simulink subsystem "controlStates"  (R2022b)
settings: Solver=VariableStepAuto  StartTime=0.0  StopTime=10.0  RelTol=1e-3
libraries: Raptor_lib x3
settings Model: Creator=serga  LastModifiedBy=serga

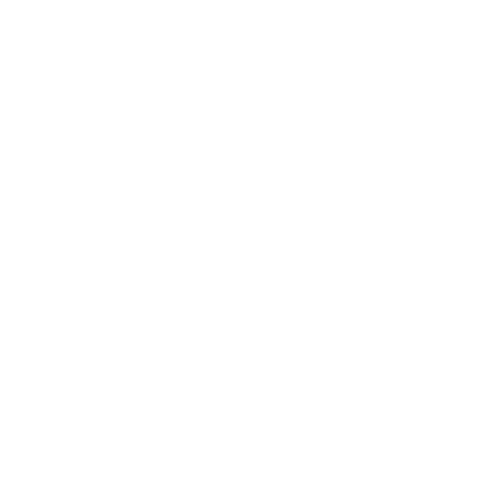
[thumbnail: Simulink's stored preview of the top-level diagram]
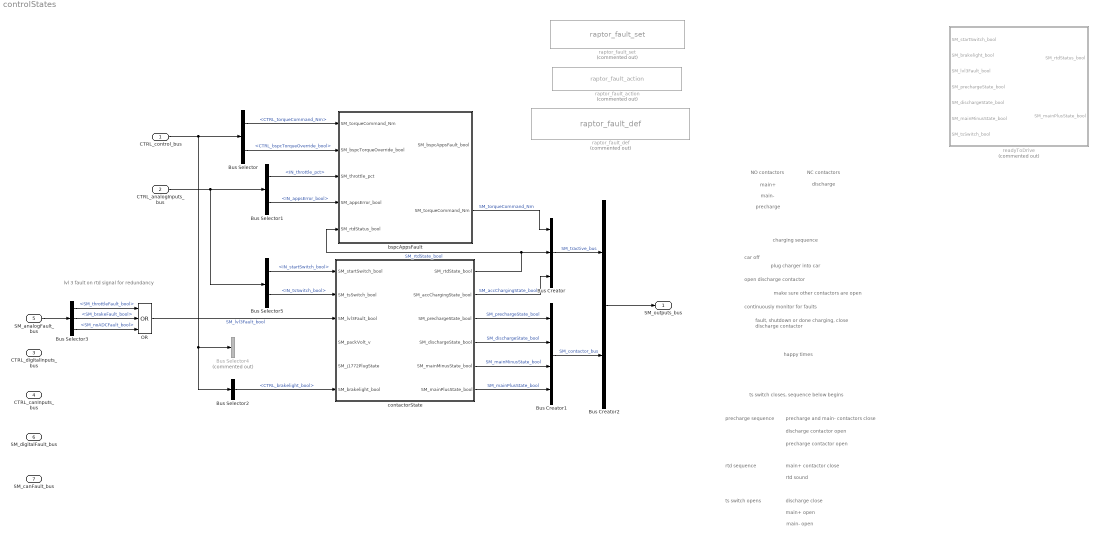
== system controlStates ==
  note: lvl 3 fault on rtd signal for redundancy
  note: ts switch closes, sequence below begins
  note: precharge sequence
  note: precharge and main- contactors close
  note: discharge contactor open
  note: NO contactors
  note: main+
  note: main-
  note: precharge
  note: precharge contactor open
  note: NC contactors
  note: discharge
  note: rtd sequence
  note: main+ contactor close
  note: rtd sound
  note: ts switch opens
  note: discharge close
  note: main+ open
  note: main- open
  note: charging sequence
  note: car off
  note: plug charger into car
  note: open discharge contactor
  note: continuously monitor for faults
  note: fault, shutdown or done charging, close discharge contactor
  note: happy times
  note: make sure other contactors are open
  CTRL_control_bus : Inport
  CTRL_analogInputs_bus : Inport  Port=2
  CTRL_digitalInputs_bus : Inport  Port=3
  CTRL_canInputs_bus : Inport  Port=4
  SM_analogFault_bus : Inport  Port=5
  SM_digitalFault_bus : Inport  Port=6
  SM_canFault_bus : Inport  Port=7
  Bus Creator : BusCreator  Inputs=3
  Bus Creator1 : BusCreator  Inputs=4
  Bus Creator2 : BusCreator  Inputs=2
  Bus Selector : BusSelector  OutputSignals=CTRL_tractive_bus.CTRL_torqueCommand_Nm,CTRL_tractive_bus.CTRL_bspcTorqueOverride_bool
  Bus Selector1 : BusSelector  OutputSignals=IN_throttle_bus.IN_throttle_pct,IN_throttle_bus.IN_appsError_bool
  Bus Selector2 : BusSelector  OutputSignals=CTRL_brake_bus.CTRL_brakelight_bool
  Bus Selector3 : BusSelector  OutputSignals=SM_lvl3AnalogFault_bus.SM_throttleFault_bool,SM_lvl3AnalogFault_bus.SM_brakeFault_bool,SM_lvl3AnalogFault_bus.SM_noADCFault_bool
  Bus Selector4 : BusSelector  Commented=on  OutputSignals=signal1,signal2
  Bus Selector5 : BusSelector  OutputSignals=IN_startSwitch_bus.IN_startSwitch_bool,IN_tsSwitch_bus.IN_tsSwitch_bool
  OR : Logic  Operator=OR  Inputs=3  IconShape=distinctive  AllPortsSameDT=off  OutDataTypeStr=boolean
  bspcAppsFault : Stateflow chart  TreatAsAtomicUnit=on
      settings: PortSchema="{\"entries\":[{\"content\":{\"sides\":[{\"content\":{\"connectorIds\":[\"In1\",\"In2\",\"In5\",\"In3\",\"In4\"]},\"type\":\"ConnectorPlacement.EquallySpacedRectSide\",\"uuid\":\"848a0214-b289-4fde-8f30-558c176c1664\"},{\"content\":{\"connectorIds\":[\"Out1\",\"Out2\"],\"side\":\"RIGHT\"},\"type\":\"ConnectorPlacement.EquallySpacedRectSide\",\"uuid\":\"0594a9c2-6fff-42f9-9aad-f57b5a6a5f51\"},{\"content\":{\"connectorIds\":[],\"side\":\"TOP\"},\"type\":\"ConnectorPlacement.EquallySpacedRectSide\",\"uuid\":\"66d9e814-45e9-4ebd-81f9-9e1bbba2abf2\"}]},\"type\":\"ConnectorPlacement.EquallySpacedConnector\",\"uuid\":\"77a7b6c4-8b57-4880-abaf-81cbc3ed0df8\"}],\"packageUris\":[\"http://schema.mathworks.com/mf0/Connector/R2020b\"],\"version\":\"1.0\"}"
  contactorState : Stateflow chart  TreatAsAtomicUnit=on
      settings: PortSchema="{\"entries\":[{\"content\":{\"sides\":[{\"content\":{\"connectorIds\":[\"In5\",\"In1\",\"In3\",\"In2\",\"In4\",\"In6\"]},\"type\":\"ConnectorPlacement.EquallySpacedRectSide\",\"uuid\":\"5a1b01df-5f74-4071-b1de-8ca561e5e723\"},{\"content\":{\"connectorIds\":[\"Out4\",\"Out6\",\"Out1\",\"Out2\",\"Out3\",\"Out5\"],\"side\":\"RIGHT\"},\"type\":\"ConnectorPlacement.EquallySpacedRectSide\",\"uuid\":\"0ef1ebc5-2a8c-458a-b0e0-8c2b473d38b4\"},{\"content\":{\"connectorIds\":[],\"side\":\"TOP\"},\"type\":\"ConnectorPlacement.EquallySpacedRectSide\",\"uuid\":\"5065868a-8688-4951-998e-140db11ca85e\"}]},\"type\":\"ConnectorPlacement.EquallySpacedConnector\",\"uuid\":\"42e1f654-1cfc-4608-be09-c21f3bede254\"}],\"packageUris\":[\"http://schema.mathworks.com/mf0/Connector/R2020b\"],\"version\":\"1.0\"}"
  raptor_fault_action : Raptor_lib/Faults/raptor_fault_action  Commented=on  actionName='myFaultAction'  calVisible=off  calAccess=1  calFunction='System | FaultManager | FaultAction'
      settings: SourceProductName=Raptor
  raptor_fault_def : Raptor_lib/Faults/raptor_fault_def  Commented=on  faultName='SM_bspcAppsFault_bool'  persist=off  sticky=off  emisRelated=off  singleTrip=off  clearMethod=Standard  xLimit=25  yLimit=50  calEnable=on  addDisable=off  calAccess=1  calFunction='System | FaultManager'
      settings: SourceProductName=Raptor
  raptor_fault_set : Raptor_lib/Faults/raptor_fault_set  Commented=on  faultSourceValues=[]  faultSource=2  faultName='myFault'  stateValues=[]  state=2  inhibitPort=0
      settings: SourceProductName=Raptor
  readyToDrive : Stateflow chart  Commented=on  TreatAsAtomicUnit=on
      settings: PortSchema="{\"entries\":[{\"content\":{\"sides\":[{\"content\":{\"connectorIds\":[\"In1\",\"In2\",\"In7\",\"In3\",\"In4\",\"In5\",\"In6\"]},\"type\":\"ConnectorPlacement.EquallySpacedRectSide\",\"uuid\":\"7a40ea6c-59dd-455f-a32c-fa2d09cb7cc1\"},{\"content\":{\"connectorIds\":[\"Out1\",\"Out2\"],\"side\":\"RIGHT\"},\"type\":\"ConnectorPlacement.EquallySpacedRectSide\",\"uuid\":\"57ddf04d-63e3-4b1a-8e75-1315c8d70976\"},{\"content\":{\"connectorIds\":[],\"side\":\"TOP\"},\"type\":\"ConnectorPlacement.EquallySpacedRectSide\",\"uuid\":\"3f096798-bb3f-4081-9c59-6b5844ba7ac4\"}]},\"type\":\"ConnectorPlacement.EquallySpacedConnector\",\"uuid\":\"b65609e6-e8f6-4a29-a634-254e4debf82f\"}],\"packageUris\":[\"http://schema.mathworks.com/mf0/Connector/R2020b\"],\"version\":\"1.0\"}"
  SM_outputs_bus : Outport
  wires:
  Bus Selector5/2 -> contactorState/1(SM_tsSwitch_bool)  "<IN_tsSwitch_bool>"
  Bus Selector5/1 -> contactorState/5(SM_startSwitch_bool)  "<IN_startSwitch_bool>"
  OR/1 -> contactorState/3(SM_lvl3Fault_bool)  "SM_lvl3Fault_bool"
  Bus Selector2/1 -> contactorState/6(SM_brakelight_bool)  "<CTRL_brakelight_bool>"
  Bus Selector1/1 -> bspcAppsFault/5(SM_throttle_pct)  "<IN_throttle_pct>"
  bspcAppsFault/2(SM_torqueCommand_Nm) -> Bus Creator/1  "SM_torqueCommand_Nm"
  contactorState/6(SM_accChargingState_bool) -> Bus Creator/3  "SM_accChargingState_bool"
  contactorState/4(SM_rtdState_bool) -> Bus Creator/2, bspcAppsFault/4(SM_rtdStatus_bool)  "SM_rtdState_bool"
  contactorState/5(SM_mainPlusState_bool) -> Bus Creator1/4  "SM_mainPlusState_bool"
  contactorState/3(SM_mainMinusState_bool) -> Bus Creator1/3  "SM_mainMinusState_bool"
  contactorState/2(SM_dischargeState_bool) -> Bus Creator1/2  "SM_dischargeState_bool"
  contactorState/1(SM_prechargeState_bool) -> Bus Creator1/1  "SM_prechargeState_bool"
  Bus Selector1/2 -> bspcAppsFault/3(SM_appsError_bool)  "<IN_appsError_bool>"
  Bus Selector/2 -> bspcAppsFault/2(SM_bspcTorqueOverride_bool)  "<CTRL_bspcTorqueOverride_bool>"
  Bus Selector/1 -> bspcAppsFault/1("SM_torqueCommand_Nm ")  "<CTRL_torqueCommand_Nm>"
  Bus Selector3/3 -> OR/3  "<SM_noADCFault_bool>"
  SM_analogFault_bus/1 -> Bus Selector3/1
  Bus Selector3/2 -> OR/2  "<SM_brakeFault_bool>"
  Bus Selector3/1 -> OR/1  "<SM_throttleFault_bool>"
  Bus Creator2/1 -> SM_outputs_bus/1
  Bus Creator1/1 -> Bus Creator2/2  "SM_contactor_bus"
  Bus Creator/1 -> Bus Creator2/1  "SM_tractive_bus"
  CTRL_control_bus/1 -> Bus Selector/1, Bus Selector2/1, Bus Selector4/1
  CTRL_analogInputs_bus/1 -> Bus Selector5/1, Bus Selector1/1

== stateflow chart controlStates/bspcAppsFault ==
  state BSPC_APPS_Fault
    during: SM_torqueCommand_Nm = 0; % set the command to 0 until proper condition is met
    en: SM_bspcAppsFault_bool = true; % create the fault variable
  note: can command torque once throttle is less than 5%
  state Normal
    en: SM_torqueCommand_Nm; % current torque command
    en: SM_bspcTorqueOverride_bool; % override flag due to brk + thr
    en: SM_throttle_pct; % for throttle pct
    en: SM_appsError_bool; % 10% disparity between thr1 + thr2
    during: SM_bspcAppsFault_bool = false;
    en: SM_torqueCommand_Nm;
    en: SM_rtdStatus_bool; % rtd state
  BSPC_APPS_Fault -> (junction 13)
  (junction 13) -> (junction 12) : [SM_throttle_pct < 5.0 ...
      | && SM_bspcTorqueOverride_bool == false ...
      | && SM_appsError_bool == false ...
      | && SM_rtdStatus_bool == true]
  (junction 11) -> BSPC_APPS_Fault
  (junction 14) -> (junction 11) : [(SM_bspcTorqueOverride_bool == true ...
      | || SM_appsError_bool == true) ...
      | && SM_rtdStatus_bool == true]
  (default) -> Normal
  Normal -> (junction 14)
  (junction 12) -> Normal
  data: SM_bspcAppsFault_bool output; SM_torqueCommand_Nm input; SM_bspcTorqueOverride_bool input; SM_appsError_bool input; SM_torqueCommand_Nm output; SM_rtdStatus_bool input; SM_throttle_pct input

== stateflow chart controlStates/contactorState ==
  note: ?
  state ChargeCircuit
    ex: SM_dischargeState_bool = false;
    ex: SM_accChargingState_bool = false;
    ex: SM_mainMinusState_bool = false;
    ex: SM_mainPlusState_bool = false;
    state ChargingStandby
    state Charging
      en: SM_dischargeState_bool = true;
      en: SM_mainPlusState_bool = true;
      en: SM_mainMinusState_bool = true;
      en: SM_accChargingState_bool = true;
    (default) -> ChargingStandby
    ChargingStandby -> Charging : [SM_j1772PlugState == 4]
    Charging -> ChargingStandby : [SM_j1772PlugState == 0 ...
        | || SM_j1772PlugState == 2 ...
        | || SM_j1772PlugState == 3]
  state ReadyToDrive
    ex: SM_rtdState_bool = false;
    % throw system out of rtd when critical error
    ex: SM_mainPlusState_bool = false;
    state RTDStandby
    state RTD
      en: SM_rtdState_bool = true; % have a boolean condition for critical sensors??
      % throw system out of rtd when critical error
      en: SM_mainPlusState_bool = true;
    note: check vehicle states to be sure car can go into rtd mode
    (default) -> RTDStandby
    RTDStandby -> RTD : [SM_tsSwitch_bool == true ...
        | && SM_prechargeState_bool == false ...
        | && SM_dischargeState_bool == true ...
        | && SM_mainMinusState_bool == true ...
        | && SM_brakelight_bool == true ...
        | && SM_startSwitch_bool == true ...
        | && SM_dischargeState_bool == true ...
        | && SM_lvl3Fault_bool == false]
  note: 240 volts from min cell voltage * 96
  note: 403 volts from max cell voltage * 96
  note: get the car out of rtd as soon as the charger is detected
  state PrechargeCircuit
    note: needs 90+% accumulator voltage, and an extra 0.5 secs for precharge to be considered complete
    note: variables change on block entry
    note: added an extra second for padding
    state PrechargeClosed % precharge is complete when the circuit contains 90+% of the total voltage
      en: SM_mainMinusState_bool = true; % close main- contactor
      en: SM_prechargeState_bool = true; % close precharge contactor
    state PrechargeComplete
      en: SM_prechargeState_bool = false; % open contactor
      en: SM_dischargeState_bool = true; % open contactor
    note: once precharging is considered to be complete, open the discharge contactor
    note: ts active when shutdown circuit receives power
    note: when ts switch is off, power to inverter should be cut
    state PrechargeOpen
      en: SM_tsSwitch_bool; % tractive system active
      en: SM_packVolt_v; % monitoring voltage on the tractive system
      % when ts is active, precharge contactor is closed
      % TSA means > 60V but I am simply using it as a trigger for precharging
      en: SM_prechargeState_bool = false; % normally open
      en: SM_mainMinusState_bool = false; % normally open
      en: SM_mainPlusState_bool = false; % normally open
      en: SM_dischargeState_bool = false; % normally closed
      % error check so contactors can close when something bas happens
      en: SM_lvl3Fault_bool;
      % grab charging data/status
      en: SM_j1772PlugState;
    note: precharge contactor should be open
    note: precharge will be disabled
    PrechargeClosed % precharge is complete when the circuit contains 90+% of the total voltage -> (junction 112) [order 1]
    (junction 112) -> (junction 110) : [SM_tsSwitch_bool == false ...
        | || SM_lvl3Fault_bool == true]
    PrechargeClosed % precharge is complete when the circuit contains 90+% of the total voltage -> PrechargeComplete [order 2] : [(duration(SM_packVolt_v >= 311) > 1.5) ...
        | && SM_lvl3Fault_bool == false]
    (junction 107) -> PrechargeClosed % precharge is complete when the circuit contains 90+% of the total voltage
    (junction 108) -> (junction 107) : [SM_tsSwitch_bool == true ...
        | && SM_lvl3Fault_bool == false]
    PrechargeComplete -> (junction 109) [commented out] : [SM_tsSwitch_bool == false  ...
        | || SM_dischargeState_bool == false ...
        | || SM_packVolt_v < 240 ...
        | || SM_packVolt_v > 403 ...
        | || SM_lvl3Fault_bool == true]
    (default) -> PrechargeOpen
    PrechargeOpen -> (junction 108)
    (junction 109) -> PrechargeOpen [commented out]
    (junction 110) -> PrechargeOpen
  PrechargeCircuit -> ChargeCircuit [order 1] : [(SM_j1772PlugState == 0 ...
      | || SM_j1772PlugState == 2 ...
      | || SM_j1772PlugState == 3 ...
      | || SM_j1772PlugState == 4)]
  ChargeCircuit -> PrechargeCircuit : [SM_j1772PlugState == 1]
  PrechargeCircuit -> ReadyToDrive [order 2] : [SM_prechargeState_bool == false ...
      | && SM_dischargeState_bool == true ...
      | && SM_mainMinusState_bool == true]
  ReadyToDrive -> PrechargeCircuit : [SM_tsSwitch_bool == false  ...
      | || SM_dischargeState_bool == false ...
      | || SM_packVolt_v < 240 ...
      | || SM_packVolt_v > 403 ...
      | || SM_lvl3Fault_bool == true ...
      | || SM_j1772PlugState == 4]
  (default) -> PrechargeCircuit
  data: SM_prechargeState_bool output; SM_dischargeState_bool output; SM_mainMinusState_bool output; SM_tsSwitch_bool input; SM_packVolt_v input; SM_lvl3Fault_bool input; SM_j1772PlugState input; SM_rtdState_bool output boolean; SM_mainPlusState_bool output; SM_startSwitch_bool input; SM_brakelight_bool input; SM_accChargingState_bool output

== stateflow chart controlStates/readyToDrive ==
  state RTD
    en: SM_rtdStatus_bool = true; % have a boolean condition for critical sensors??
    % throw system out of rtd when critical error
    en: SM_mainPlusState_bool = true;
  note: check vehicle states to be sure car can go into rtd mode
  state Standby
    en: SM_tsSwitch_bool % ts active status
    en: SM_prechargeState_bool; % first RTD action
    en: SM_brakelight_bool; % used for mechancal brake actuation - second RTD action
    en: SM_startSwitch_bool; % third RTD action
    % check critical component status
    en: SM_dischargeState_bool; % make it impossible to conflict with precharging
    en: SM_mainMinusState_bool; % make it impossible to conflict with precharging
    %
    en: SM_mainPlusState_bool = false;
    en: SM_rtdStatus_bool = false;
    %
    en: SM_lvl3Fault_bool;
  RTD -> (junction 14)
  (junction 14) -> (junction 12) : [SM_tsSwitch_bool == false ...
      | || SM_lvl3Fault_bool == true]
  (junction 11) -> RTD
  (junction 4) -> (junction 11) : [SM_tsSwitch_bool == true ...
      | && SM_prechargeState_bool == false ...
      | && SM_dischargeState_bool == true ...
      | && SM_mainMinusState_bool == true ...
      | && SM_brakelight_bool == true ...
      | && SM_startSwitch_bool == true ...
      | && SM_dischargeState_bool == true ...
      | && SM_lvl3Fault_bool == false]
  (default) -> Standby
  Standby -> (junction 4)
  (junction 12) -> Standby
  data: SM_startSwitch_bool input; SM_brakelight_bool input; SM_rtdStatus_bool output; SM_prechargeState_bool input; SM_dischargeState_bool input; SM_mainMinusState_bool input; SM_mainPlusState_bool output; SM_tsSwitch_bool input; SM_lvl3Fault_bool input
